simulink subsystem "MotorMixingAlgorithm"  (R2025a)
settings: Solver=VariableStepAuto  StartTime=0.0  StopTime=10.0  RelTol=1e-3
undefined symbols (not defined in the file): b, d_t, l
settings Model: Creator=tobia  LastModifiedBy=dma

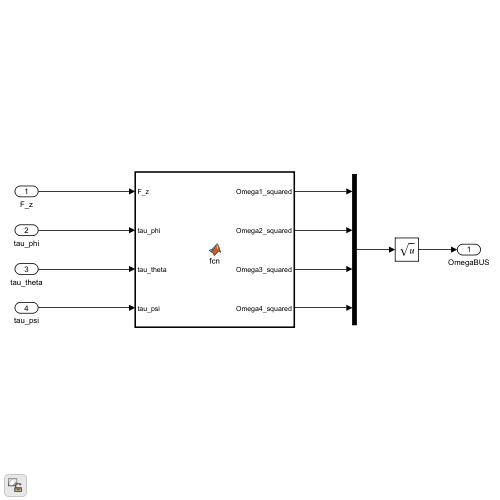
[thumbnail: Simulink's stored preview of the top-level diagram]
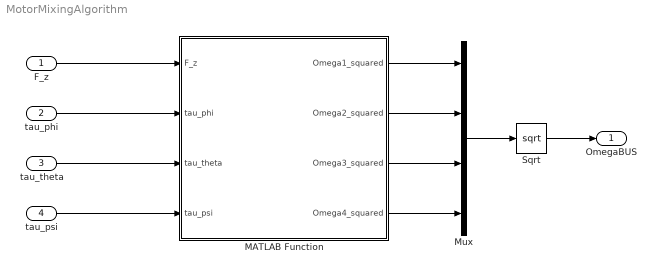
== system MotorMixingAlgorithm ==
  F_z : Inport
  tau_phi : Inport  Port=2
  tau_theta : Inport  Port=3
  tau_psi : Inport  Port=4
  MATLAB Function : MATLAB Function  TreatAsAtomicUnit=on
  Mux : Mux
  Sqrt : Sqrt
  OmegaBUS : Outport
  wires:
  tau_phi/1 -> MATLAB Function/2(tau_phi)
  F_z/1 -> MATLAB Function/1(F_z)
  tau_theta/1 -> MATLAB Function/3(tau_theta)
  tau_psi/1 -> MATLAB Function/4(tau_psi)
  MATLAB Function/1(Omega1_squared) -> Mux/1
  MATLAB Function/2(Omega2_squared) -> Mux/2
  MATLAB Function/3(Omega3_squared) -> Mux/3
  MATLAB Function/4(Omega4_squared) -> Mux/4
  Mux/1 -> Sqrt/1
  Sqrt/1 -> OmegaBUS/1

== matlab function MotorMixingAlgorithm/MATLAB Function ==
  data: F_z input; Omega1_squared output; Omega2_squared output; Omega3_squared output; Omega4_squared output; tau_phi input; tau_theta input; tau_psi input; b parameter; l parameter; d_t parameter
function [Omega1_squared, Omega2_squared, Omega3_squared, Omega4_squared]  = fcn(F_z, tau_phi, tau_theta, tau_psi, b, l, d_t)
Omega1_squared = F_z - tau_theta - tau_psi;
Omega2_squared = F_z - tau_phi + tau_psi;
Omega3_squared = F_z + tau_theta - tau_psi;
Omega4_squared = F_z + tau_phi + tau_psi;

%{
Omega1_squared = 1/(4*b)*F_z - 1/(2*b*l)*tau_theta - 1/(4*d_t)*tau_psi;
Omega2_squared = 1/(4*b)*F_z - 1/(2*b*l)*tau_phi + 1/(4*d_t)*tau_psi;
Omega3_squared = 1/(4*b)*F_z + 1/(2*b*l)*tau_theta - 1/(4*d_t)*tau_psi;
Omega4_squared = 1/(4*b)*F_z + 1/(2*b*l)*tau_phi + 1/(4*d_t)*tau_psi;

disp('Altitude')
display(1/(4*b)*F_z)
disp("theta")
display(1/(2*b*l)*tau_theta)
disp("phi")
display(1/(2*b*l)*tau_phi)
display(1/(4*d_t)*tau_psi)

    + phi (roll) -        
                           
        
        3↻   
        |                     +
  ↺4 ---o--- 2↺  theta (pitch)
        |                     _
        1↻   
                    

Legend:
+/- = sign of introduced angle
↻  = clockwise rotation
↺  = counterclockwise rotation
o  = center of quadcopter
Numbers 1–4 = rotor indices
https://cookierobotics.com/066/
%}
